simulink model "Model_TranslationEngine64"  (R2022b)
settings: Solver=FixedStepDiscrete  StartTime=0.0  StopTime=5  RelTol=1e-3  EnableMultiTasking=on
InitFcn:
  | % Initialize model
  | ModelSettings=BTConfig.GetModelSettings();
  | 
  | ModelSettings.Validate();
  | 
  | ModelInit;
  | 
  | 
  | % load library data
  | GainLibrary_data;
  | % Load saved values from partition process
  | CapturedConstMask.LoadMapFromFile(bdroot)
StartFcn:
  | % make sure all the simulated RTC requests are found
  | %RTC_SIM_OBJ.ValidateREQs();
undefined symbols (not defined in the file or in its folder): AA, BPLP, Column, NumHFRefBPF, NumHFRefLPF, NumMusicChannels, Row, VolumeMuteConfig
libraries: TuneVar x925, TOP x490, FeaturePath x111, CapturedConstLib x52
(part 2 of 34)

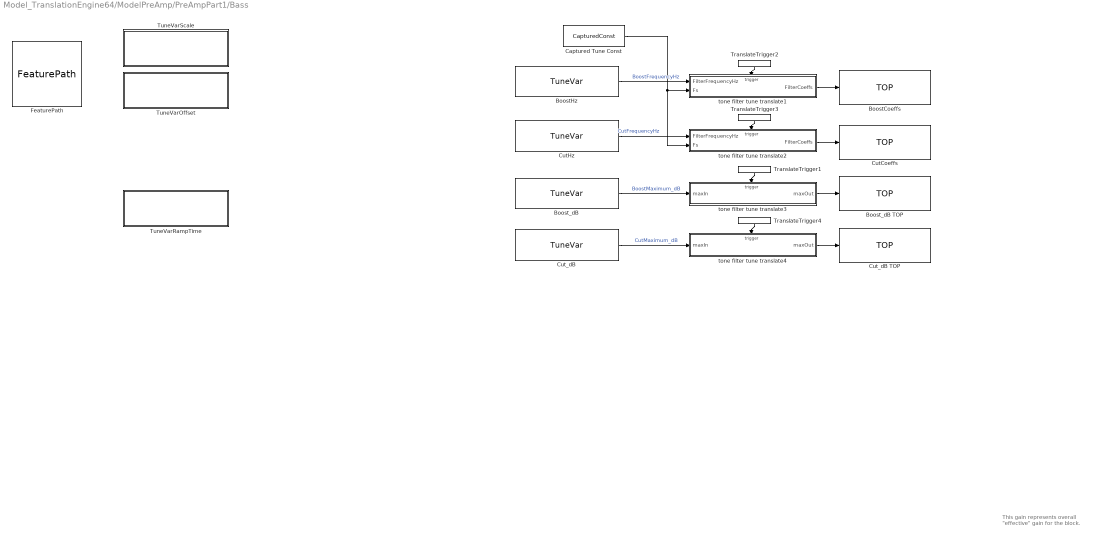
== system Model_TranslationEngine64/ModelPreAmp/PreAmpPart1/Bass ==
  note: This gain represents overall
      | "effective" gain for the block.
  BoostCoeffs : TOP/TOP  TriggerInit=[-490 -218 -340 -162]  TopName=BoostCoeffs  DataTypeOut=single  BankNumber=Config.BankNumber  PreOverlay=false  PostOverlay=false  Role=Automatic
      settings: SourceProductName=Bose Talaria
  BoostHz : TuneVar/TuneVar  Description=Indicates the 'corner frequency' of the target frequency band for the 'Boost' filter.  TuneName=BoostFrequencyHz  SpecifyMaxSize=off  VariableDim=1 (Row)  MaxSize=[1 1]  TunabilityNumber=1  MinValue=[]  MaxValue=[]  TriggerInit=[-1025 -225 -855 -175]  MaskValue=Config.DefaultBoostHz
      settings: SourceProductName=Bose Talaria
  Boost_dB : TuneVar/TuneVar  Description=Indicates the maximum impact in dB for the tone boost. This value must be positive. A negative boost impact would imply a gain cut instead!  TuneName=BoostMaximum_dB  SpecifyMaxSize=off  VariableDim=1 (Row)  MaxSize=[1 1]  TunabilityNumber=1  MinValue=[0]  MaxValue=[]  TriggerInit=[-1025 -40 -855 10]  MaskValue=Config.DefaultBoostDb
      settings: SourceProductName=Bose Talaria
  Boost_dB TOP : TOP/TOP  TriggerInit=[-490 -43 -340 13]  TopName=BoostMaximum_dB  DataTypeOut=single  BankNumber=Config.BankNumber  PreOverlay=false  PostOverlay=false  Role=Automatic
      settings: SourceProductName=Bose Talaria
  Captured Tune Const : CapturedConstLib/CapturedConst  TriggerInit=[-945 -293 -845 -257]  Role=Automatic
      settings: SourceProductName=Bose Talaria
  CutCoeffs : TOP/TOP  TriggerInit=[-490 -128 -340 -72]  TopName=CutCoeffs  DataTypeOut=single  BankNumber=Config.BankNumber  PreOverlay=false  PostOverlay=false  Role=Automatic
      settings: SourceProductName=Bose Talaria
  CutHz : TuneVar/TuneVar  Description=Indicates the 'corner frequency' of the target frequency band for the 'Cut' filter.  TuneName=CutFrequencyHz  SpecifyMaxSize=off  VariableDim=1 (Row)  MaxSize=[1 1]  TunabilityNumber=1  MinValue=[]  MaxValue=[]  TriggerInit=[-1025 -135 -855 -85]  MaskValue=Config.DefaultCutHz
      settings: SourceProductName=Bose Talaria
  Cut_dB : TuneVar/TuneVar  Description=Indicates the maximum impact in dB for the tone cut. This value must be positive. A negative cut impact would imply a gain boost instead!  TuneName=CutMaximum_dB  SpecifyMaxSize=off  VariableDim=1 (Row)  MaxSize=[1 1]  TunabilityNumber=1  MinValue=[0]  MaxValue=[]  TriggerInit=[-1025 45 -855 95]  MaskValue=Config.DefaultCutDb
      settings: SourceProductName=Bose Talaria
  Cut_dB TOP : TOP/TOP  TriggerInit=[-490 42 -340 98]  TopName=CutMaximum_dB  DataTypeOut=single  BankNumber=Config.BankNumber  PreOverlay=false  PostOverlay=false  Role=Automatic
      settings: SourceProductName=Bose Talaria
  FeaturePath : FeaturePath/FeaturePath  FeatureName=Bass  IsGroup=off  GroupNumber=-1  IsModule=off  TriggerInit=[-1855 -266 -1740 -159]
      settings: SourceProductName=Bose Talaria
  TranslateTrigger1 : TuneVar/TranslateTrigger  TriggerInit=[-657 -60 -603 -50]
      settings: SourceProductName=Bose Talaria
  TranslateTrigger2 : TuneVar/TranslateTrigger  TriggerInit=[-657 -235 -603 -225]
      settings: SourceProductName=Bose Talaria
  TranslateTrigger3 : TuneVar/TranslateTrigger  TriggerInit=[-657 -145 -603 -135]
      settings: SourceProductName=Bose Talaria
  TranslateTrigger4 : TuneVar/TranslateTrigger  TriggerInit=[-657 25 -603 35]
      settings: SourceProductName=Bose Talaria
  TuneVarOffset : Subsystem  Description=Offset represents the midpoint of the index range, which separates the 'boost' indices from the 'cut' indices.  mask(Talaria Trivial Tune TOP){TriggerInit=[-1670 -213 -1500 -157], TopName=Offset, TuneName=Offset, DataTypeOut=single, MaskValue=Config.DefaultOffset, TunabilityNumber=1, MinValue=[], MaxValue=[], BankNumber=Config.BankNumber, PreOverlay=false, PostOverlay=false, UseSameName=on}
      mask prompts: TriggerInit "Hidden: MoveFcn redraw"; TopName "Name:"; TuneName "Name of TuneVar:"; DataTypeOut "Data type:"; MaskValue "Default Value:"; TunabilityNumber "Tunability:"; MinValue "Min Value:"; MaxValue "Max Value:"; BankNumber "Target memory bank number:"; PreOverlay "Requires pre-overlay action:"; PostOverlay "Requires post-overlay action:"; UseSameName "Use same name for tune variable and TOP"
      mask help: The TuneTOP block encapsultes a Target Overlay Parameter, a Tune Variable, and a Trivial Translation between them.
      mask init:
      | [ok,activeTopPath,activeTunePath] = TuneTOP_Mask.Init(gcbh);
      settings: MoveFcn=TuneTOP_Mask.CB_TriggerInit(gcbh);
      mask Callback TriggerInit: TuneTOP_Mask.CB_TriggerInit(gcbh);
      mask TypeOptions TopName: TOP/TopName
      mask TypeOptions TuneName: Tune Variable/TuneName
      mask TypeOptions DataTypeOut: TOP/DataTypeOut
      mask TypeOptions MaskValue: Tune Variable/MaskValue
      mask TypeOptions TunabilityNumber: Tune Variable/TunabilityNumber
      mask Callback TunabilityNumber: TuneVarMask.CB_TunabilityNumber(gcbh);
      mask TypeOptions MinValue: Tune Variable/MinValue
      mask TypeOptions MaxValue: Tune Variable/MaxValue
      mask TypeOptions BankNumber: TOP/BankNumber
      mask TypeOptions PreOverlay: TOP/PreOverlay
      mask TypeOptions PostOverlay: TOP/PostOverlay
      mask Callback UseSameName: TuneTOP_Mask.CB_UseSameName(gcbh);
      mask DialogControl toolPanel Prompt: Tuning Tool Hints
      mask DialogControl DescriptionGroup Prompt: Description
      mask DialogControl EditDescription Prompt: Edit Description
      mask DialogControl EditDescription Callback: TuneTOP_Mask.CB_EditDescription(gcbh);
      mask DialogControl TunabilityText Prompt: Easy: Changes nearly every tuning.
      mask DialogControl AdvancedPanel Prompt: Advanced
      mask DialogControl ConvertToFullTranslation Prompt: Irreversible conversion to full translation
      mask DialogControl ConvertToFullTranslation Callback: TuneTOP_Mask.CB_ConvertToFullTranslation(gcbh);
      mask DialogControl ErrorContainer Prompt: Error Messages
      mask Display:
      | % retrieve icon definition
      | [path,w,h] = TuneTOP_Mask.Icon();
      | 
      | % retrieve the block's pixel size
      | pos = get(gcbh,'position');
      | bw = pos(3) - pos(1);
      | bh = pos(4) - pos(2);
      | 
      | % draw centered icon
      | xAdj = bw/2 - w/2 + 5;
      | yAdj = bh/2 - h/2 + 4;
      | for i=1:length(path)
      | 	patch(path(i).x+xAdj, path(i).y+yAdj, path(i).rgb);
      | end
      | 
      | % show the top name or an X
      | if (exist('ok','var') && ok)
      | 	text(bw*0.5, bh*0.2, activeTopPath, 'horizontalAlignment', 'center');
      | 	patch(0,0,[1 1 1]);
      | 	patch(bw,bh,[1 1 1]);
      | else
      | 	tx=bw*0.03;
      | 	ty=bh*0.03;
      | 	patch([0 tx bw bw-tx], [ty 0 bh-ty bh], [1 0 0]);
      | 	patch([0 bw-tx bw tx], [bh-ty 0 ty bh], [1 0 0]);
      | end
  TuneVarRampTime : Subsystem  Description=This is the default ramp time that will be used if the RTC message has a '0' for both ramp time and ramp rate.  mask(Talaria Trivial Tune TOP){TriggerInit=[-1670 -18 -1500 38], TopName=ramptime, TuneName=ramptime, DataTypeOut=single, MaskValue=30, TunabilityNumber=1, MinValue=1, MaxValue=100000, BankNumber=0, PreOverlay=false, PostOverlay=false, UseSameName=on}
      mask prompts: TriggerInit "Hidden: MoveFcn redraw"; TopName "Name:"; TuneName "Name of TuneVar:"; DataTypeOut "Data type:"; MaskValue "Default Value:"; TunabilityNumber "Tunability:"; MinValue "Min Value:"; MaxValue "Max Value:"; BankNumber "Target memory bank number:"; PreOverlay "Requires pre-overlay action:"; PostOverlay "Requires post-overlay action:"; UseSameName "Use same name for tune variable and TOP"
      mask help: The TuneTOP block encapsultes a Target Overlay Parameter, a Tune Variable, and a Trivial Translation between them.
      mask init:
      | [ok,activeTopPath,activeTunePath] = TuneTOP_Mask.Init(gcbh);
      settings: MoveFcn=TuneTOP_Mask.CB_TriggerInit(gcbh);
      mask Callback TriggerInit: TuneTOP_Mask.CB_TriggerInit(gcbh);
      mask TypeOptions TopName: TOP/TopName
      mask TypeOptions TuneName: Tune Variable/TuneName
      mask TypeOptions DataTypeOut: TOP/DataTypeOut
      mask TypeOptions MaskValue: Tune Variable/MaskValue
      mask TypeOptions TunabilityNumber: Tune Variable/TunabilityNumber
      mask Callback TunabilityNumber: TuneVarMask.CB_TunabilityNumber(gcbh);
      mask TypeOptions MinValue: Tune Variable/MinValue
      mask TypeOptions MaxValue: Tune Variable/MaxValue
      mask TypeOptions BankNumber: TOP/BankNumber
      mask TypeOptions PreOverlay: TOP/PreOverlay
      mask TypeOptions PostOverlay: TOP/PostOverlay
      mask Callback UseSameName: TuneTOP_Mask.CB_UseSameName(gcbh);
      mask DialogControl toolPanel Prompt: Tuning Tool Hints
      mask DialogControl DescriptionGroup Prompt: Description
      mask DialogControl EditDescription Prompt: Edit Description
      mask DialogControl EditDescription Callback: TuneTOP_Mask.CB_EditDescription(gcbh);
      mask DialogControl TunabilityText Prompt: Easy: Changes nearly every tuning.
      mask DialogControl AdvancedPanel Prompt: Advanced
      mask DialogControl ConvertToFullTranslation Prompt: Irreversible conversion to full translation
      mask DialogControl ConvertToFullTranslation Callback: TuneTOP_Mask.CB_ConvertToFullTranslation(gcbh);
      mask DialogControl ErrorContainer Prompt: Error Messages
      mask Display:
      | % retrieve icon definition
      | [path,w,h] = TuneTOP_Mask.Icon();
      | 
      | % retrieve the block's pixel size
      | pos = get(gcbh,'position');
      | bw = pos(3) - pos(1);
      | bh = pos(4) - pos(2);
      | 
      | % draw centered icon
      | xAdj = bw/2 - w/2 + 5;
      | yAdj = bh/2 - h/2 + 4;
      | for i=1:length(path)
      | 	patch(path(i).x+xAdj, path(i).y+yAdj, path(i).rgb);
      | end
      | 
      | % show the top name or an X
      | if (exist('ok','var') && ok)
      | 	text(bw*0.5, bh*0.2, activeTopPath, 'horizontalAlignment', 'center');
      | 	patch(0,0,[1 1 1]);
      | 	patch(bw,bh,[1 1 1]);
      | else
      | 	tx=bw*0.03;
      | 	ty=bh*0.03;
      | 	patch([0 tx bw bw-tx], [ty 0 bh-ty bh], [1 0 0]);
      | 	patch([0 bw-tx bw tx], [bh-ty 0 ty bh], [1 0 0]);
      | end
  TuneVarScale : Subsystem  Description=Scale is used to normalize the linear gain to a value between +/- 1. The range (0,1] represents a boost while the range [-1,0) represents a cut. We use the number of available indices in each range (mapped to gain values between [-1,1]) as the denominator for normalization, i.e. as the 'Scale'.  mask(Talaria Trivial Tune TOP){TriggerInit=[-1670 -283 -1500 -227], TopName=Scale, TuneName=Scale, DataTypeOut=single, MaskValue=Config.DefaultScale, TunabilityNumber=1, MinValue=[], MaxValue=[], BankNumber=Config.BankNumber, PreOverlay=false, PostOverlay=false, UseSameName=on}
      mask prompts: TriggerInit "Hidden: MoveFcn redraw"; TopName "Name:"; TuneName "Name of TuneVar:"; DataTypeOut "Data type:"; MaskValue "Default Value:"; TunabilityNumber "Tunability:"; MinValue "Min Value:"; MaxValue "Max Value:"; BankNumber "Target memory bank number:"; PreOverlay "Requires pre-overlay action:"; PostOverlay "Requires post-overlay action:"; UseSameName "Use same name for tune variable and TOP"
      mask help: The TuneTOP block encapsultes a Target Overlay Parameter, a Tune Variable, and a Trivial Translation between them.
      mask init:
      | [ok,activeTopPath,activeTunePath] = TuneTOP_Mask.Init(gcbh);
      settings: MoveFcn=TuneTOP_Mask.CB_TriggerInit(gcbh);
      mask Callback TriggerInit: TuneTOP_Mask.CB_TriggerInit(gcbh);
      mask TypeOptions TopName: TOP/TopName
      mask TypeOptions TuneName: Tune Variable/TuneName
      mask TypeOptions DataTypeOut: TOP/DataTypeOut
      mask TypeOptions MaskValue: Tune Variable/MaskValue
      mask TypeOptions TunabilityNumber: Tune Variable/TunabilityNumber
      mask Callback TunabilityNumber: TuneVarMask.CB_TunabilityNumber(gcbh);
      mask TypeOptions MinValue: Tune Variable/MinValue
      mask TypeOptions MaxValue: Tune Variable/MaxValue
      mask TypeOptions BankNumber: TOP/BankNumber
      mask TypeOptions PreOverlay: TOP/PreOverlay
      mask TypeOptions PostOverlay: TOP/PostOverlay
      mask Callback UseSameName: TuneTOP_Mask.CB_UseSameName(gcbh);
      mask DialogControl toolPanel Prompt: Tuning Tool Hints
      mask DialogControl DescriptionGroup Prompt: Description
      mask DialogControl EditDescription Prompt: Edit Description
      mask DialogControl EditDescription Callback: TuneTOP_Mask.CB_EditDescription(gcbh);
      mask DialogControl TunabilityText Prompt: Easy: Changes nearly every tuning.
      mask DialogControl AdvancedPanel Prompt: Advanced
      mask DialogControl ConvertToFullTranslation Prompt: Irreversible conversion to full translation
      mask DialogControl ConvertToFullTranslation Callback: TuneTOP_Mask.CB_ConvertToFullTranslation(gcbh);
      mask DialogControl ErrorContainer Prompt: Error Messages
      mask Display:
      | % retrieve icon definition
      | [path,w,h] = TuneTOP_Mask.Icon();
      | 
      | % retrieve the block's pixel size
      | pos = get(gcbh,'position');
      | bw = pos(3) - pos(1);
      | bh = pos(4) - pos(2);
      | 
      | % draw centered icon
      | xAdj = bw/2 - w/2 + 5;
      | yAdj = bh/2 - h/2 + 4;
      | for i=1:length(path)
      | 	patch(path(i).x+xAdj, path(i).y+yAdj, path(i).rgb);
      | end
      | 
      | % show the top name or an X
      | if (exist('ok','var') && ok)
      | 	text(bw*0.5, bh*0.2, activeTopPath, 'horizontalAlignment', 'center');
      | 	patch(0,0,[1 1 1]);
      | 	patch(bw,bh,[1 1 1]);
      | else
      | 	tx=bw*0.03;
      | 	ty=bh*0.03;
      | 	patch([0 tx bw bw-tx], [ty 0 bh-ty bh], [1 0 0]);
      | 	patch([0 bw-tx bw tx], [bh-ty 0 ty bh], [1 0 0]);
      | end
  tone filter tune translate1 : MATLAB Function  TreatAsAtomicUnit=on  mask{MaskFilterType=Config.FilterType}
      mask prompts: MaskFilterType "Filter type"
  tone filter tune translate2 : MATLAB Function  TreatAsAtomicUnit=on  mask{MaskFilterType=Config.FilterType}
      mask prompts: MaskFilterType "Filter type"
  tone filter tune translate3 : MATLAB Function  TreatAsAtomicUnit=on
  tone filter tune translate4 : MATLAB Function  TreatAsAtomicUnit=on
  wires:
  TranslateTrigger4/1 -> tone filter tune translate4/Trigger
  TranslateTrigger1/1 -> tone filter tune translate3/Trigger
  Captured Tune Const/1 -> tone filter tune translate1/2(Fs), tone filter tune translate2/2(Fs)
  tone filter tune translate4/1(maxOut) -> Cut_dB TOP/1
  Cut_dB/1 -> tone filter tune translate4/1(maxIn)  "CutMaximum_dB"
  tone filter tune translate3/1(maxOut) -> Boost_dB TOP/1
  Boost_dB/1 -> tone filter tune translate3/1(maxIn)  "BoostMaximum_dB"
  tone filter tune translate2/1(FilterCoeffs) -> CutCoeffs/1
  tone filter tune translate1/1(FilterCoeffs) -> BoostCoeffs/1
  CutHz/1 -> tone filter tune translate2/1(FilterFrequencyHz)  "CutFrequencyHz"
  TranslateTrigger3/1 -> tone filter tune translate2/Trigger
  BoostHz/1 -> tone filter tune translate1/1(FilterFrequencyHz)  "BoostFrequencyHz"
  TranslateTrigger2/1 -> tone filter tune translate1/Trigger

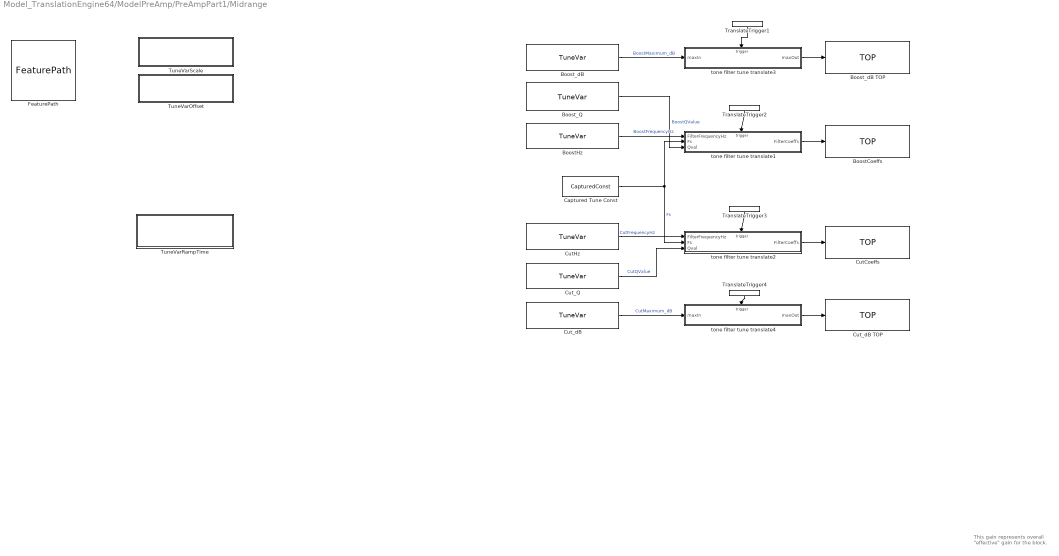
== system Model_TranslationEngine64/ModelPreAmp/PreAmpPart1/Midrange ==
  note: This gain represents overall
      | "effective" gain for the block.
  BoostCoeffs : TOP/TOP  TriggerInit=[1775 237 1925 293]  TopName=BoostCoeffs  DataTypeOut=single  BankNumber=Config.BankNumber  PreOverlay=false  PostOverlay=false  Role=Automatic
      settings: SourceProductName=Bose Talaria
  BoostHz : TuneVar/TuneVar  Description=Indicates the 'center frequency' of the target frequency band for the 'Boost' filter.  TuneName=BoostFrequencyHz  SpecifyMaxSize=off  VariableDim=1 (Row)  MaxSize=[1 1]  TunabilityNumber=1  MinValue=[]  MaxValue=[]  TriggerInit=[1240 232 1405 278]  MaskValue=Config.DefaultBoostHz
      settings: SourceProductName=Bose Talaria
  Boost_Q : TuneVar/TuneVar  Description=Value represents the width of the frequency band for the 'Boost' filter.  TuneName=BoostQValue  SpecifyMaxSize=off  VariableDim=1 (Row)  MaxSize=[1 1]  TunabilityNumber=1  MinValue=[]  MaxValue=[]  TriggerInit=[1240 160 1405 210]  MaskValue=Config.DefaultBoostq
      settings: SourceProductName=Bose Talaria
  Boost_dB : TuneVar/TuneVar  Description=Indicates the maximum impact in dB for the tone boost. This value must be positive. A negative boost impact would imply a gain cut instead!  TuneName=BoostMaximum_dB  SpecifyMaxSize=off  VariableDim=1 (Row)  MaxSize=[1 1]  TunabilityNumber=1  MinValue=[0]  MaxValue=[]  TriggerInit=[1240 92 1405 138]  MaskValue=Config.DefaultBoostDb
      settings: SourceProductName=Bose Talaria
  Boost_dB TOP : TOP/TOP  TriggerInit=[1775 87 1925 143]  TopName=BoostMaximum_dB  DataTypeOut=single  BankNumber=Config.BankNumber  PreOverlay=false  PostOverlay=false  Role=Automatic
      settings: SourceProductName=Bose Talaria
  Captured Tune Const : CapturedConstLib/CapturedConst  TriggerInit=[1305 327 1405 363]  Role=Automatic
      settings: SourceProductName=Bose Talaria
  CutCoeffs : TOP/TOP  TriggerInit=[1775 417 1925 473]  TopName=CutCoeffs  DataTypeOut=single  BankNumber=Config.BankNumber  PreOverlay=false  PostOverlay=false  Role=Automatic
      settings: SourceProductName=Bose Talaria
  CutHz : TuneVar/TuneVar  Description=Indicates the 'center frequency' of the target frequency band for the 'Cut' filter.  TuneName=CutFrequencyHz  SpecifyMaxSize=off  VariableDim=1 (Row)  MaxSize=[1 1]  TunabilityNumber=1  MinValue=[]  MaxValue=[]  TriggerInit=[1240 412 1405 458]  MaskValue=Config.DefaultCutHz
      settings: SourceProductName=Bose Talaria
  Cut_Q : TuneVar/TuneVar  Description=Value represents the width of the frequency band for the 'Cut' filter.  TuneName=CutQValue  SpecifyMaxSize=off  VariableDim=1 (Row)  MaxSize=[1 1]  TunabilityNumber=1  MinValue=[0]  MaxValue=[]  TriggerInit=[1240 482 1405 528]  MaskValue=Config.DefaultCutq
      settings: SourceProductName=Bose Talaria
  Cut_dB : TuneVar/TuneVar  Description=Indicates the maximum impact in dB for the tone cut. This value must be positive. A negative cut impact would imply a gain boost instead!  TuneName=CutMaximum_dB  SpecifyMaxSize=off  VariableDim=1 (Row)  MaxSize=[1 1]  TunabilityNumber=1  MinValue=[0]  MaxValue=[]  TriggerInit=[1240 552 1405 598]  MaskValue=Config.DefaultCutDb
      settings: SourceProductName=Bose Talaria
  Cut_dB TOP : TOP/TOP  TriggerInit=[1775 547 1925 603]  TopName=CutMaximum_dB  DataTypeOut=single  BankNumber=Config.BankNumber  PreOverlay=false  PostOverlay=false  Role=Automatic
      settings: SourceProductName=Bose Talaria
  FeaturePath : FeaturePath/FeaturePath  FeatureName=Midrange  IsGroup=off  GroupNumber=-1  IsModule=off  TriggerInit=[320 84 435 191]
      settings: SourceProductName=Bose Talaria
  TranslateTrigger1 : TuneVar/TranslateTrigger  TriggerInit=[1608 50 1662 60]
      settings: SourceProductName=Bose Talaria
  TranslateTrigger2 : TuneVar/TranslateTrigger  TriggerInit=[1603 200 1657 210]
      settings: SourceProductName=Bose Talaria
  TranslateTrigger3 : TuneVar/TranslateTrigger  TriggerInit=[1603 380 1657 390]
      settings: SourceProductName=Bose Talaria
  TranslateTrigger4 : TuneVar/TranslateTrigger  TriggerInit=[1603 530 1657 540]
      settings: SourceProductName=Bose Talaria
  TuneVarOffset : Subsystem  Description=Offset represents the midpoint of the index range, which separates the 'boost' indices from the 'cut' indices.  mask(Talaria Trivial Tune TOP){TriggerInit=[550 147 715 193], TopName=Offset, TuneName=Offset, DataTypeOut=single, MaskValue=Config.DefaultDefaultOffset, TunabilityNumber=1, MinValue=[], MaxValue=[], BankNumber=0, PreOverlay=false, PostOverlay=false, UseSameName=on}
      mask prompts: TriggerInit "Hidden: MoveFcn redraw"; TopName "Name:"; TuneName "Name of TuneVar:"; DataTypeOut "Data type:"; MaskValue "Default Value:"; TunabilityNumber "Tunability:"; MinValue "Min Value:"; MaxValue "Max Value:"; BankNumber "Target memory bank number:"; PreOverlay "Requires pre-overlay action:"; PostOverlay "Requires post-overlay action:"; UseSameName "Use same name for tune variable and TOP"
      mask help: The TuneTOP block encapsultes a Target Overlay Parameter, a Tune Variable, and a Trivial Translation between them.
      mask init:
      | [ok,activeTopPath,activeTunePath] = TuneTOP_Mask.Init(gcbh);
      settings: MoveFcn=TuneTOP_Mask.CB_TriggerInit(gcbh);
      mask Callback TriggerInit: TuneTOP_Mask.CB_TriggerInit(gcbh);
      mask TypeOptions TopName: TOP/TopName
      mask TypeOptions TuneName: Tune Variable/TuneName
      mask TypeOptions DataTypeOut: TOP/DataTypeOut
      mask TypeOptions MaskValue: Tune Variable/MaskValue
      mask TypeOptions TunabilityNumber: Tune Variable/TunabilityNumber
      mask Callback TunabilityNumber: TuneVarMask.CB_TunabilityNumber(gcbh);
      mask TypeOptions MinValue: Tune Variable/MinValue
      mask TypeOptions MaxValue: Tune Variable/MaxValue
      mask TypeOptions BankNumber: TOP/BankNumber
      mask TypeOptions PreOverlay: TOP/PreOverlay
      mask TypeOptions PostOverlay: TOP/PostOverlay
      mask Callback UseSameName: TuneTOP_Mask.CB_UseSameName(gcbh);
      mask DialogControl toolPanel Prompt: Tuning Tool Hints
      mask DialogControl DescriptionGroup Prompt: Description
      mask DialogControl EditDescription Prompt: Edit Description
      mask DialogControl EditDescription Callback: TuneTOP_Mask.CB_EditDescription(gcbh);
      mask DialogControl TunabilityText Prompt: Easy: Changes nearly every tuning.
      mask DialogControl AdvancedPanel Prompt: Advanced
      mask DialogControl ConvertToFullTranslation Prompt: Irreversible conversion to full translation
      mask DialogControl ConvertToFullTranslation Callback: TuneTOP_Mask.CB_ConvertToFullTranslation(gcbh);
      mask DialogControl ErrorContainer Prompt: Error Messages
      mask Display:
      | % retrieve icon definition
      | [path,w,h] = TuneTOP_Mask.Icon();
      | 
      | % retrieve the block's pixel size
      | pos = get(gcbh,'position');
      | bw = pos(3) - pos(1);
      | bh = pos(4) - pos(2);
      | 
      | % draw centered icon
      | xAdj = bw/2 - w/2 + 5;
      | yAdj = bh/2 - h/2 + 4;
      | for i=1:length(path)
      | 	patch(path(i).x+xAdj, path(i).y+yAdj, path(i).rgb);
      | end
      | 
      | % show the top name or an X
      | if (exist('ok','var') && ok)
      | 	text(bw*0.5, bh*0.2, activeTopPath, 'horizontalAlignment', 'center');
      | 	patch(0,0,[1 1 1]);
      | 	patch(bw,bh,[1 1 1]);
      | else
      | 	tx=bw*0.03;
      | 	ty=bh*0.03;
      | 	patch([0 tx bw bw-tx], [ty 0 bh-ty bh], [1 0 0]);
      | 	patch([0 bw-tx bw tx], [bh-ty 0 ty bh], [1 0 0]);
      | end
  TuneVarRampTime : Subsystem  Description=This is the default ramp time that will be used if the RTC message has a '0' for both ramp time and ramp rate.  mask(Talaria Trivial Tune TOP){TriggerInit=[545 397 715 453], TopName=RampTime, TuneName=RampTime, DataTypeOut=single, MaskValue=30, TunabilityNumber=1, MinValue=1, MaxValue=100000, BankNumber=0, PreOverlay=false, PostOverlay=false, UseSameName=on}
      mask prompts: TriggerInit "Hidden: MoveFcn redraw"; TopName "Name:"; TuneName "Name of TuneVar:"; DataTypeOut "Data type:"; MaskValue "Default Value:"; TunabilityNumber "Tunability:"; MinValue "Min Value:"; MaxValue "Max Value:"; BankNumber "Target memory bank number:"; PreOverlay "Requires pre-overlay action:"; PostOverlay "Requires post-overlay action:"; UseSameName "Use same name for tune variable and TOP"
      mask help: The TuneTOP block encapsultes a Target Overlay Parameter, a Tune Variable, and a Trivial Translation between them.
      mask init:
      | [ok,activeTopPath,activeTunePath] = TuneTOP_Mask.Init(gcbh);
      settings: MoveFcn=TuneTOP_Mask.CB_TriggerInit(gcbh);
      mask Callback TriggerInit: TuneTOP_Mask.CB_TriggerInit(gcbh);
      mask TypeOptions TopName: TOP/TopName
      mask TypeOptions TuneName: Tune Variable/TuneName
      mask TypeOptions DataTypeOut: TOP/DataTypeOut
      mask TypeOptions MaskValue: Tune Variable/MaskValue
      mask TypeOptions TunabilityNumber: Tune Variable/TunabilityNumber
      mask Callback TunabilityNumber: TuneVarMask.CB_TunabilityNumber(gcbh);
      mask TypeOptions MinValue: Tune Variable/MinValue
      mask TypeOptions MaxValue: Tune Variable/MaxValue
      mask TypeOptions BankNumber: TOP/BankNumber
      mask TypeOptions PreOverlay: TOP/PreOverlay
      mask TypeOptions PostOverlay: TOP/PostOverlay
      mask Callback UseSameName: TuneTOP_Mask.CB_UseSameName(gcbh);
      mask DialogControl toolPanel Prompt: Tuning Tool Hints
      mask DialogControl DescriptionGroup Prompt: Description
      mask DialogControl EditDescription Prompt: Edit Description
      mask DialogControl EditDescription Callback: TuneTOP_Mask.CB_EditDescription(gcbh);
      mask DialogControl TunabilityText Prompt: Easy: Changes nearly every tuning.
      mask DialogControl AdvancedPanel Prompt: Advanced
      mask DialogControl ConvertToFullTranslation Prompt: Irreversible conversion to full translation
      mask DialogControl ConvertToFullTranslation Callback: TuneTOP_Mask.CB_ConvertToFullTranslation(gcbh);
      mask DialogControl ErrorContainer Prompt: Error Messages
      mask Display:
      | % retrieve icon definition
      | [path,w,h] = TuneTOP_Mask.Icon();
      | 
      | % retrieve the block's pixel size
      | pos = get(gcbh,'position');
      | bw = pos(3) - pos(1);
      | bh = pos(4) - pos(2);
      | 
      | % draw centered icon
      | xAdj = bw/2 - w/2 + 5;
      | yAdj = bh/2 - h/2 + 4;
      | for i=1:length(path)
      | 	patch(path(i).x+xAdj, path(i).y+yAdj, path(i).rgb);
      | end
      | 
      | % show the top name or an X
      | if (exist('ok','var') && ok)
      | 	text(bw*0.5, bh*0.2, activeTopPath, 'horizontalAlignment', 'center');
      | 	patch(0,0,[1 1 1]);
      | 	patch(bw,bh,[1 1 1]);
      | else
      | 	tx=bw*0.03;
      | 	ty=bh*0.03;
      | 	patch([0 tx bw bw-tx], [ty 0 bh-ty bh], [1 0 0]);
      | 	patch([0 bw-tx bw tx], [bh-ty 0 ty bh], [1 0 0]);
      | end
  TuneVarScale : Subsystem  Description=Scale is used to normalize the linear gain to a value between +/- 1. The range (0,1] represents a boost while the range [-1,0) represents a cut. We use the number of available indices in each range (mapped to gain values between [-1,1]) as the denominator for normalization, i.e. as the 'Scale'.  mask(Talaria Trivial Tune TOP){TriggerInit=[550 81 715 129], TopName=Scale, TuneName=Scale, DataTypeOut=single, MaskValue=Config.DefaultDefaultScale, TunabilityNumber=1, MinValue=[], MaxValue=[], BankNumber=0, PreOverlay=false, PostOverlay=false, UseSameName=on}
      mask prompts: TriggerInit "Hidden: MoveFcn redraw"; TopName "Name:"; TuneName "Name of TuneVar:"; DataTypeOut "Data type:"; MaskValue "Default Value:"; TunabilityNumber "Tunability:"; MinValue "Min Value:"; MaxValue "Max Value:"; BankNumber "Target memory bank number:"; PreOverlay "Requires pre-overlay action:"; PostOverlay "Requires post-overlay action:"; UseSameName "Use same name for tune variable and TOP"
      mask help: The TuneTOP block encapsultes a Target Overlay Parameter, a Tune Variable, and a Trivial Translation between them.
      mask init:
      | [ok,activeTopPath,activeTunePath] = TuneTOP_Mask.Init(gcbh);
      settings: MoveFcn=TuneTOP_Mask.CB_TriggerInit(gcbh);
      mask Callback TriggerInit: TuneTOP_Mask.CB_TriggerInit(gcbh);
      mask TypeOptions TopName: TOP/TopName
      mask TypeOptions TuneName: Tune Variable/TuneName
      mask TypeOptions DataTypeOut: TOP/DataTypeOut
      mask TypeOptions MaskValue: Tune Variable/MaskValue
      mask TypeOptions TunabilityNumber: Tune Variable/TunabilityNumber
      mask Callback TunabilityNumber: TuneVarMask.CB_TunabilityNumber(gcbh);
      mask TypeOptions MinValue: Tune Variable/MinValue
      mask TypeOptions MaxValue: Tune Variable/MaxValue
      mask TypeOptions BankNumber: TOP/BankNumber
      mask TypeOptions PreOverlay: TOP/PreOverlay
      mask TypeOptions PostOverlay: TOP/PostOverlay
      mask Callback UseSameName: TuneTOP_Mask.CB_UseSameName(gcbh);
      mask DialogControl toolPanel Prompt: Tuning Tool Hints
      mask DialogControl DescriptionGroup Prompt: Description
      mask DialogControl EditDescription Prompt: Edit Description
      mask DialogControl EditDescription Callback: TuneTOP_Mask.CB_EditDescription(gcbh);
      mask DialogControl TunabilityText Prompt: Easy: Changes nearly every tuning.
      mask DialogControl AdvancedPanel Prompt: Advanced
      mask DialogControl ConvertToFullTranslation Prompt: Irreversible conversion to full translation
      mask DialogControl ConvertToFullTranslation Callback: TuneTOP_Mask.CB_ConvertToFullTranslation(gcbh);
      mask DialogControl ErrorContainer Prompt: Error Messages
      mask Display:
      | % retrieve icon definition
      | [path,w,h] = TuneTOP_Mask.Icon();
      | 
      | % retrieve the block's pixel size
      | pos = get(gcbh,'position');
      | bw = pos(3) - pos(1);
      | bh = pos(4) - pos(2);
      | 
      | % draw centered icon
      | xAdj = bw/2 - w/2 + 5;
      | yAdj = bh/2 - h/2 + 4;
      | for i=1:length(path)
      | 	patch(path(i).x+xAdj, path(i).y+yAdj, path(i).rgb);
      | end
      | 
      | % show the top name or an X
      | if (exist('ok','var') && ok)
      | 	text(bw*0.5, bh*0.2, activeTopPath, 'horizontalAlignment', 'center');
      | 	patch(0,0,[1 1 1]);
      | 	patch(bw,bh,[1 1 1]);
      | else
      | 	tx=bw*0.03;
      | 	ty=bh*0.03;
      | 	patch([0 tx bw bw-tx], [ty 0 bh-ty bh], [1 0 0]);
      | 	patch([0 bw-tx bw tx], [bh-ty 0 ty bh], [1 0 0]);
      | end
  tone filter tune translate1 : MATLAB Function  TreatAsAtomicUnit=on
  tone filter tune translate2 : MATLAB Function  TreatAsAtomicUnit=on
  tone filter tune translate3 : MATLAB Function  TreatAsAtomicUnit=on
  tone filter tune translate4 : MATLAB Function  TreatAsAtomicUnit=on
  wires:
  tone filter tune translate2/1(FilterCoeffs) -> CutCoeffs/1
  TranslateTrigger1/1 -> tone filter tune translate3/Trigger
  Cut_Q/1 -> tone filter tune translate2/3(Qval)  "CutQValue"
  TranslateTrigger4/1 -> tone filter tune translate4/Trigger
  BoostHz/1 -> tone filter tune translate1/1(FilterFrequencyHz)  "BoostFrequencyHz"
  TranslateTrigger2/1 -> tone filter tune translate1/Trigger
  TranslateTrigger3/1 -> tone filter tune translate2/Trigger
  tone filter tune translate4/1(maxOut) -> Cut_dB TOP/1
  Captured Tune Const/1 -> tone filter tune translate2/2(Fs), tone filter tune translate1/2(Fs)  "Fs"
  tone filter tune translate1/1(FilterCoeffs) -> BoostCoeffs/1
  Cut_dB/1 -> tone filter tune translate4/1(maxIn)  "CutMaximum_dB"
  Boost_dB/1 -> tone filter tune translate3/1(maxIn)  "BoostMaximum_dB"
  tone filter tune translate3/1(maxOut) -> Boost_dB TOP/1
  Boost_Q/1 -> tone filter tune translate1/3(Qval)  "BoostQValue"
  CutHz/1 -> tone filter tune translate2/1(FilterFrequencyHz)  "CutFrequencyHz"

== system Model_TranslationEngine64/ModelPreAmp/PreAmpPart1/NEARPreAmp ==
  FixedAttenuator : Subsystem  mask{Config=Config.FixedAttenuator}
      mask prompts: Config "FixedAttenuatorConfig"
      mask init:
      | blkh=gcbh;
      | Config=BTConfig.Assert(blkh,Config);
      | 
      | Config.Validate();
      | Config.DoMaskInit(blkh);
      mask DialogControl ClassContainer Prompt: Fixed Attenuator Class Instance
  Monoizer : Subsystem  mask(Monoizer){Config=Config.Monoizer}
      mask prompts: Config "MonoizerConfig"
      mask help:
      | This mask allows the setting of parameters for the Monoizer model.
      | Model parameters are set by a class instance in the base workspace.
      |
      | See 'Help' for details.
      mask init:
      | blkh=gcbh;
      | Config=BTConfig.Assert(blkh,Config);
      | 
      | Config.Validate();
      | Config.DoMaskInit(blkh);
      mask Help:
      | Defining model parameters:
      | The model parameters are set by the conents of an instance of MonoizerClass.m.
      | 
      | To set model parameters:
      | 1-Create an instance of MonoizerClass.m in the base workspace.
      | 2-In the model mask, set the 'Class instance' parameter to the name of the class instance in the base workspace.
  MusicLimiter : Subsystem  mask(MusicLimiter){Config=Config.MusicLimiter}
      mask prompts: Config "MusicLimiterConfig"
      mask help:
      | This mask allows the setting of parameters for the MusicLimiter model.
      | Model parameters are set by a class instance in the base workspace.
      |
      | See 'Help' for details.
      mask init:
      | blkh=gcbh;
      | Config=BTConfig.Assert(blkh,Config);
      | 
      | Config.Validate();
      | Config.DoMaskInit(blkh);
      mask Help:
      | Defining model parameters:
      | The model parameters are set by the conents of an instance of MusicLimiterClass.m.
      | 
      | To set model parameters:
      | 1-Create an instance of MusicLimiterClass.m in the base workspace.
      | 2-In the model mask, set the 'Class instance' parameter to the name of the class instance in the base workspace.

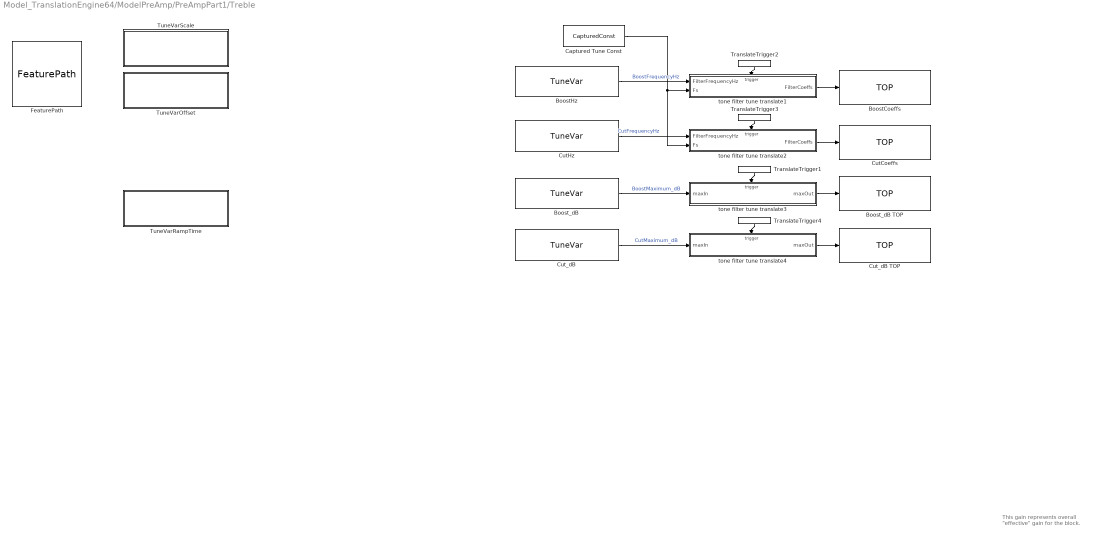
== system Model_TranslationEngine64/ModelPreAmp/PreAmpPart1/Treble ==
  note: This gain represents overall
      | "effective" gain for the block.
  BoostCoeffs : TOP/TOP  TriggerInit=[-490 -218 -340 -162]  TopName=BoostCoeffs  DataTypeOut=single  BankNumber=Config.BankNumber  PreOverlay=false  PostOverlay=false  Role=Automatic
      settings: SourceProductName=Bose Talaria
  BoostHz : TuneVar/TuneVar  Description=Indicates the 'corner frequency' of the target frequency band for the 'Boost' filter.  TuneName=BoostFrequencyHz  SpecifyMaxSize=off  VariableDim=1 (Row)  MaxSize=[1 1]  TunabilityNumber=1  MinValue=[]  MaxValue=[]  TriggerInit=[-1025 -225 -855 -175]  MaskValue=Config.DefaultBoostHz
      settings: SourceProductName=Bose Talaria
  Boost_dB : TuneVar/TuneVar  Description=Indicates the maximum impact in dB for the tone boost. This value must be positive. A negative boost impact would imply a gain cut instead!  TuneName=BoostMaximum_dB  SpecifyMaxSize=off  VariableDim=1 (Row)  MaxSize=[1 1]  TunabilityNumber=1  MinValue=[0]  MaxValue=[]  TriggerInit=[-1025 -40 -855 10]  MaskValue=Config.DefaultBoostDb
      settings: SourceProductName=Bose Talaria
  Boost_dB TOP : TOP/TOP  TriggerInit=[-490 -43 -340 13]  TopName=BoostMaximum_dB  DataTypeOut=single  BankNumber=Config.BankNumber  PreOverlay=false  PostOverlay=false  Role=Automatic
      settings: SourceProductName=Bose Talaria
  Captured Tune Const : CapturedConstLib/CapturedConst  TriggerInit=[-945 -293 -845 -257]  Role=Automatic
      settings: SourceProductName=Bose Talaria
  CutCoeffs : TOP/TOP  TriggerInit=[-490 -128 -340 -72]  TopName=CutCoeffs  DataTypeOut=single  BankNumber=Config.BankNumber  PreOverlay=false  PostOverlay=false  Role=Automatic
      settings: SourceProductName=Bose Talaria
  CutHz : TuneVar/TuneVar  Description=Indicates the 'corner frequency' of the target frequency band for the 'Cut' filter.  TuneName=CutFrequencyHz  SpecifyMaxSize=off  VariableDim=1 (Row)  MaxSize=[1 1]  TunabilityNumber=1  MinValue=[]  MaxValue=[]  TriggerInit=[-1025 -135 -855 -85]  MaskValue=Config.DefaultCutHz
      settings: SourceProductName=Bose Talaria
  Cut_dB : TuneVar/TuneVar  Description=Indicates the maximum impact in dB for the tone cut. This value must be positive. A negative cut impact would imply a gain boost instead!  TuneName=CutMaximum_dB  SpecifyMaxSize=off  VariableDim=1 (Row)  MaxSize=[1 1]  TunabilityNumber=1  MinValue=[0]  MaxValue=[]  TriggerInit=[-1025 45 -855 95]  MaskValue=Config.DefaultCutDb
      settings: SourceProductName=Bose Talaria
  Cut_dB TOP : TOP/TOP  TriggerInit=[-490 42 -340 98]  TopName=CutMaximum_dB  DataTypeOut=single  BankNumber=Config.BankNumber  PreOverlay=false  PostOverlay=false  Role=Automatic
      settings: SourceProductName=Bose Talaria
  FeaturePath : FeaturePath/FeaturePath  FeatureName=Treble  IsGroup=off  GroupNumber=-1  IsModule=off  TriggerInit=[-1855 -266 -1740 -159]
      settings: SourceProductName=Bose Talaria
  TranslateTrigger1 : TuneVar/TranslateTrigger  TriggerInit=[-657 -60 -603 -50]
      settings: SourceProductName=Bose Talaria
  TranslateTrigger2 : TuneVar/TranslateTrigger  TriggerInit=[-657 -235 -603 -225]
      settings: SourceProductName=Bose Talaria
  TranslateTrigger3 : TuneVar/TranslateTrigger  TriggerInit=[-657 -145 -603 -135]
      settings: SourceProductName=Bose Talaria
  TranslateTrigger4 : TuneVar/TranslateTrigger  TriggerInit=[-657 25 -603 35]
      settings: SourceProductName=Bose Talaria
  TuneVarOffset : Subsystem  Description=Offset represents the midpoint of the index range, which separates the 'boost' indices from the 'cut' indices.  mask(Talaria Trivial Tune TOP){TriggerInit=[-1670 -213 -1500 -157], TopName=Offset, TuneName=Offset, DataTypeOut=single, MaskValue=Config.DefaultOffset, TunabilityNumber=1, MinValue=[], MaxValue=[], BankNumber=Config.BankNumber, PreOverlay=false, PostOverlay=false, UseSameName=on}
      mask prompts: TriggerInit "Hidden: MoveFcn redraw"; TopName "Name:"; TuneName "Name of TuneVar:"; DataTypeOut "Data type:"; MaskValue "Default Value:"; TunabilityNumber "Tunability:"; MinValue "Min Value:"; MaxValue "Max Value:"; BankNumber "Target memory bank number:"; PreOverlay "Requires pre-overlay action:"; PostOverlay "Requires post-overlay action:"; UseSameName "Use same name for tune variable and TOP"
      mask help: The TuneTOP block encapsultes a Target Overlay Parameter, a Tune Variable, and a Trivial Translation between them.
      mask init:
      | [ok,activeTopPath,activeTunePath] = TuneTOP_Mask.Init(gcbh);
      settings: MoveFcn=TuneTOP_Mask.CB_TriggerInit(gcbh);
      mask Callback TriggerInit: TuneTOP_Mask.CB_TriggerInit(gcbh);
      mask TypeOptions TopName: TOP/TopName
      mask TypeOptions TuneName: Tune Variable/TuneName
      mask TypeOptions DataTypeOut: TOP/DataTypeOut
      mask TypeOptions MaskValue: Tune Variable/MaskValue
      mask TypeOptions TunabilityNumber: Tune Variable/TunabilityNumber
      mask Callback TunabilityNumber: TuneVarMask.CB_TunabilityNumber(gcbh);
      mask TypeOptions MinValue: Tune Variable/MinValue
      mask TypeOptions MaxValue: Tune Variable/MaxValue
      mask TypeOptions BankNumber: TOP/BankNumber
      mask TypeOptions PreOverlay: TOP/PreOverlay
      mask TypeOptions PostOverlay: TOP/PostOverlay
      mask Callback UseSameName: TuneTOP_Mask.CB_UseSameName(gcbh);
      mask DialogControl toolPanel Prompt: Tuning Tool Hints
      mask DialogControl DescriptionGroup Prompt: Description
      mask DialogControl EditDescription Prompt: Edit Description
      mask DialogControl EditDescription Callback: TuneTOP_Mask.CB_EditDescription(gcbh);
      mask DialogControl TunabilityText Prompt: Easy: Changes nearly every tuning.
      mask DialogControl AdvancedPanel Prompt: Advanced
      mask DialogControl ConvertToFullTranslation Prompt: Irreversible conversion to full translation
      mask DialogControl ConvertToFullTranslation Callback: TuneTOP_Mask.CB_ConvertToFullTranslation(gcbh);
      mask DialogControl ErrorContainer Prompt: Error Messages
      mask Display:
      | % retrieve icon definition
      | [path,w,h] = TuneTOP_Mask.Icon();
      | 
      | % retrieve the block's pixel size
      | pos = get(gcbh,'position');
      | bw = pos(3) - pos(1);
      | bh = pos(4) - pos(2);
      | 
      | % draw centered icon
      | xAdj = bw/2 - w/2 + 5;
      | yAdj = bh/2 - h/2 + 4;
      | for i=1:length(path)
      | 	patch(path(i).x+xAdj, path(i).y+yAdj, path(i).rgb);
      | end
      | 
      | % show the top name or an X
      | if (exist('ok','var') && ok)
      | 	text(bw*0.5, bh*0.2, activeTopPath, 'horizontalAlignment', 'center');
      | 	patch(0,0,[1 1 1]);
      | 	patch(bw,bh,[1 1 1]);
      | else
      | 	tx=bw*0.03;
      | 	ty=bh*0.03;
      | 	patch([0 tx bw bw-tx], [ty 0 bh-ty bh], [1 0 0]);
      | 	patch([0 bw-tx bw tx], [bh-ty 0 ty bh], [1 0 0]);
      | end
  TuneVarRampTime : Subsystem  Description=This is the default ramp time that will be used if the RTC message has a '0' for both ramp time and ramp rate.  mask(Talaria Trivial Tune TOP){TriggerInit=[-1670 -18 -1500 38], TopName=ramptime, TuneName=ramptime, DataTypeOut=single, MaskValue=30, TunabilityNumber=1, MinValue=1, MaxValue=100000, BankNumber=0, PreOverlay=false, PostOverlay=false, UseSameName=on}
      mask prompts: TriggerInit "Hidden: MoveFcn redraw"; TopName "Name:"; TuneName "Name of TuneVar:"; DataTypeOut "Data type:"; MaskValue "Default Value:"; TunabilityNumber "Tunability:"; MinValue "Min Value:"; MaxValue "Max Value:"; BankNumber "Target memory bank number:"; PreOverlay "Requires pre-overlay action:"; PostOverlay "Requires post-overlay action:"; UseSameName "Use same name for tune variable and TOP"
      mask help: The TuneTOP block encapsultes a Target Overlay Parameter, a Tune Variable, and a Trivial Translation between them.
      mask init:
      | [ok,activeTopPath,activeTunePath] = TuneTOP_Mask.Init(gcbh);
      settings: MoveFcn=TuneTOP_Mask.CB_TriggerInit(gcbh);
      mask Callback TriggerInit: TuneTOP_Mask.CB_TriggerInit(gcbh);
      mask TypeOptions TopName: TOP/TopName
      mask TypeOptions TuneName: Tune Variable/TuneName
      mask TypeOptions DataTypeOut: TOP/DataTypeOut
      mask TypeOptions MaskValue: Tune Variable/MaskValue
      mask TypeOptions TunabilityNumber: Tune Variable/TunabilityNumber
      mask Callback TunabilityNumber: TuneVarMask.CB_TunabilityNumber(gcbh);
      mask TypeOptions MinValue: Tune Variable/MinValue
      mask TypeOptions MaxValue: Tune Variable/MaxValue
      mask TypeOptions BankNumber: TOP/BankNumber
      mask TypeOptions PreOverlay: TOP/PreOverlay
      mask TypeOptions PostOverlay: TOP/PostOverlay
      mask Callback UseSameName: TuneTOP_Mask.CB_UseSameName(gcbh);
      mask DialogControl toolPanel Prompt: Tuning Tool Hints
      mask DialogControl DescriptionGroup Prompt: Description
      mask DialogControl EditDescription Prompt: Edit Description
      mask DialogControl EditDescription Callback: TuneTOP_Mask.CB_EditDescription(gcbh);
      mask DialogControl TunabilityText Prompt: Easy: Changes nearly every tuning.
      mask DialogControl AdvancedPanel Prompt: Advanced
      mask DialogControl ConvertToFullTranslation Prompt: Irreversible conversion to full translation
      mask DialogControl ConvertToFullTranslation Callback: TuneTOP_Mask.CB_ConvertToFullTranslation(gcbh);
      mask DialogControl ErrorContainer Prompt: Error Messages
      mask Display:
      | % retrieve icon definition
      | [path,w,h] = TuneTOP_Mask.Icon();
      | 
      | % retrieve the block's pixel size
      | pos = get(gcbh,'position');
      | bw = pos(3) - pos(1);
      | bh = pos(4) - pos(2);
      | 
      | % draw centered icon
      | xAdj = bw/2 - w/2 + 5;
      | yAdj = bh/2 - h/2 + 4;
      | for i=1:length(path)
      | 	patch(path(i).x+xAdj, path(i).y+yAdj, path(i).rgb);
      | end
      | 
      | % show the top name or an X
      | if (exist('ok','var') && ok)
      | 	text(bw*0.5, bh*0.2, activeTopPath, 'horizontalAlignment', 'center');
      | 	patch(0,0,[1 1 1]);
      | 	patch(bw,bh,[1 1 1]);
      | else
      | 	tx=bw*0.03;
      | 	ty=bh*0.03;
      | 	patch([0 tx bw bw-tx], [ty 0 bh-ty bh], [1 0 0]);
      | 	patch([0 bw-tx bw tx], [bh-ty 0 ty bh], [1 0 0]);
      | end
  TuneVarScale : Subsystem  Description=Scale is used to normalize the linear gain to a value between +/- 1. The range (0,1] represents a boost while the range [-1,0) represents a cut. We use the number of available indices in each range (mapped to gain values between [-1,1]) as the denominator for normalization, i.e. as the 'Scale'.  mask(Talaria Trivial Tune TOP){TriggerInit=[-1670 -283 -1500 -227], TopName=Scale, TuneName=Scale, DataTypeOut=single, MaskValue=Config.DefaultScale, TunabilityNumber=1, MinValue=[], MaxValue=[], BankNumber=Config.BankNumber, PreOverlay=false, PostOverlay=false, UseSameName=on}
      mask prompts: TriggerInit "Hidden: MoveFcn redraw"; TopName "Name:"; TuneName "Name of TuneVar:"; DataTypeOut "Data type:"; MaskValue "Default Value:"; TunabilityNumber "Tunability:"; MinValue "Min Value:"; MaxValue "Max Value:"; BankNumber "Target memory bank number:"; PreOverlay "Requires pre-overlay action:"; PostOverlay "Requires post-overlay action:"; UseSameName "Use same name for tune variable and TOP"
      mask help: The TuneTOP block encapsultes a Target Overlay Parameter, a Tune Variable, and a Trivial Translation between them.
      mask init:
      | [ok,activeTopPath,activeTunePath] = TuneTOP_Mask.Init(gcbh);
      settings: MoveFcn=TuneTOP_Mask.CB_TriggerInit(gcbh);
      mask Callback TriggerInit: TuneTOP_Mask.CB_TriggerInit(gcbh);
      mask TypeOptions TopName: TOP/TopName
      mask TypeOptions TuneName: Tune Variable/TuneName
      mask TypeOptions DataTypeOut: TOP/DataTypeOut
      mask TypeOptions MaskValue: Tune Variable/MaskValue
      mask TypeOptions TunabilityNumber: Tune Variable/TunabilityNumber
      mask Callback TunabilityNumber: TuneVarMask.CB_TunabilityNumber(gcbh);
      mask TypeOptions MinValue: Tune Variable/MinValue
      mask TypeOptions MaxValue: Tune Variable/MaxValue
      mask TypeOptions BankNumber: TOP/BankNumber
      mask TypeOptions PreOverlay: TOP/PreOverlay
      mask TypeOptions PostOverlay: TOP/PostOverlay
      mask Callback UseSameName: TuneTOP_Mask.CB_UseSameName(gcbh);
      mask DialogControl toolPanel Prompt: Tuning Tool Hints
      mask DialogControl DescriptionGroup Prompt: Description
      mask DialogControl EditDescription Prompt: Edit Description
      mask DialogControl EditDescription Callback: TuneTOP_Mask.CB_EditDescription(gcbh);
      mask DialogControl TunabilityText Prompt: Easy: Changes nearly every tuning.
      mask DialogControl AdvancedPanel Prompt: Advanced
      mask DialogControl ConvertToFullTranslation Prompt: Irreversible conversion to full translation
      mask DialogControl ConvertToFullTranslation Callback: TuneTOP_Mask.CB_ConvertToFullTranslation(gcbh);
      mask DialogControl ErrorContainer Prompt: Error Messages
      mask Display:
      | % retrieve icon definition
      | [path,w,h] = TuneTOP_Mask.Icon();
      | 
      | % retrieve the block's pixel size
      | pos = get(gcbh,'position');
      | bw = pos(3) - pos(1);
      | bh = pos(4) - pos(2);
      | 
      | % draw centered icon
      | xAdj = bw/2 - w/2 + 5;
      | yAdj = bh/2 - h/2 + 4;
      | for i=1:length(path)
      | 	patch(path(i).x+xAdj, path(i).y+yAdj, path(i).rgb);
      | end
      | 
      | % show the top name or an X
      | if (exist('ok','var') && ok)
      | 	text(bw*0.5, bh*0.2, activeTopPath, 'horizontalAlignment', 'center');
      | 	patch(0,0,[1 1 1]);
      | 	patch(bw,bh,[1 1 1]);
      | else
      | 	tx=bw*0.03;
      | 	ty=bh*0.03;
      | 	patch([0 tx bw bw-tx], [ty 0 bh-ty bh], [1 0 0]);
      | 	patch([0 bw-tx bw tx], [bh-ty 0 ty bh], [1 0 0]);
      | end
  tone filter tune translate1 : MATLAB Function  TreatAsAtomicUnit=on  mask{MaskFilterType=Config.FilterType}
      mask prompts: MaskFilterType "Filter type"
  tone filter tune translate2 : MATLAB Function  TreatAsAtomicUnit=on  mask{MaskFilterType=Config.FilterType}
      mask prompts: MaskFilterType "Filter type"
  tone filter tune translate3 : MATLAB Function  TreatAsAtomicUnit=on
  tone filter tune translate4 : MATLAB Function  TreatAsAtomicUnit=on
  wires:
  TranslateTrigger4/1 -> tone filter tune translate4/Trigger
  TranslateTrigger1/1 -> tone filter tune translate3/Trigger
  Captured Tune Const/1 -> tone filter tune translate1/2(Fs), tone filter tune translate2/2(Fs)
  tone filter tune translate4/1(maxOut) -> Cut_dB TOP/1
  Cut_dB/1 -> tone filter tune translate4/1(maxIn)  "CutMaximum_dB"
  tone filter tune translate3/1(maxOut) -> Boost_dB TOP/1
  Boost_dB/1 -> tone filter tune translate3/1(maxIn)  "BoostMaximum_dB"
  tone filter tune translate2/1(FilterCoeffs) -> CutCoeffs/1
  tone filter tune translate1/1(FilterCoeffs) -> BoostCoeffs/1
  CutHz/1 -> tone filter tune translate2/1(FilterFrequencyHz)  "CutFrequencyHz"
  TranslateTrigger3/1 -> tone filter tune translate2/Trigger
  BoostHz/1 -> tone filter tune translate1/1(FilterFrequencyHz)  "BoostFrequencyHz"
  TranslateTrigger2/1 -> tone filter tune translate1/Trigger
